simulink model "BBK_client_2006b"  (Simulink 6.5)
settings: Solver=ode3  StartTime=0.0  StopTime=Inf  FixedStep=base_dT  MaxStep=0.01  RelTol=1e-3
values from neighbouring files (symbols this model uses):
  base_dT = Simulink.Parameter    [InternetBBKInit.m]
libraries: simulink x1
settings Model: Creator=akshart  LastModifiedBy=me-dspace
settings DebuggingCC: SignalResolutionControl=UseLocalSettings  FcnCallInpInsideContextMsg=Enable All  StrictBusMsg=ErrorLevel1
settings HardwareCC: TargetHWDeviceType=32-bit Generic
settings CodeAppCC: CustomSymbolStrType=$N$R$M_T
settings GRTTargetCC: ExtModeInterfaceLevel=Level1
settings ConfigurationSet: Description=SimMechanics 2G

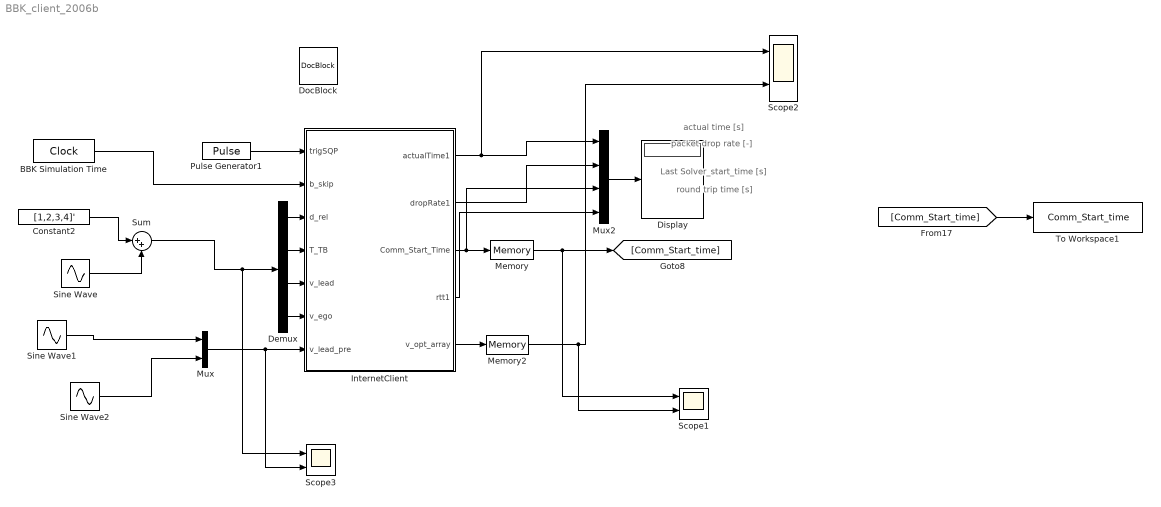
== system BBK_client_2006b ==
  note: actual time [s]
  note: packet drop rate [-]
  note: Last Solver_start_time [s]
  note: round trip time [s]
  BBK Simulation Time : DigitalClock  SampleTime=base_dT
  Constant2 : Constant  Value=[1,2,3,4]'
  Demux : Demux
  Display : Display
  DocBlock : simulink/Model-Wide Utilities/DocBlock  DocumentType=Text
  InternetClient : Subsystem
      mask Type: 20-sim 4.6 S-Function block
      mask Description:
      | This block is generated by the 20-sim Matlab Code Generator.
      | 
      | * look under the mask to get information on the ports
      | * press Help for more detailed information
      | * the parameters of this block are:
      mask Help:
      | This block is generated by the 20-sim Matlab Code Generator<br>
      | The block parameters are:<br><blockquote></blockquote>
      | Generated at:<br>
      | <blockquote><b>date:  </b>June 14, 2017<br>
      | <b>time:  </b>4:16:43 PM<br></blockquote>
      | From the following 20-sim model:<br>
      | <blockquote><b>submodel:  </b>InternetServer<br>
      | <b>model:  </b>export to Simulink - UM<br>
      | <b>file:  </b>C:\Users\Tulga Ersal\Desktop\For Xueru\export to Simulink - UM.emx<br>
      | <b>experiment:  </b>C:\Users\Tulga Ersal\Desktop\For Xueru\export to Simulink - UM.emx<br></blockquote>
      | Using the following 20-sim license:<br>
      | <blockquote><b>user:  </b>The University of Michigan<br>
      | <b>from:  </b>20-sim 4.6 Student License<br>
      | <b>build: </b>4.6.1.6898<br></blockquote>
  Memory : Memory  InheritSampleTime=on  LinearizeAsDelay=on
  Memory2 : Memory  X0=zeros(2,1)  InheritSampleTime=on  LinearizeAsDelay=on
  Mux : Mux  Inputs=2
  Mux2 : Mux
  Pulse Generator1 : DiscretePulseGenerator  PulseType=Time based  Period=1  PulseWidth=20  SampleTime=base_dT
  Scope1 : Scope  NumInputPorts=2
      settings: YMin=-0.25~-0.5  YMax=2.25~4.5
  Scope2 : Scope  NumInputPorts=2
      settings: YMin=-3.575~-5  YMax=32.175~5
  Scope3 : Scope  NumInputPorts=2
      settings: YMin=-1.71028~-1.71028  YMax=15.39249~15.39249  SaveName=ScopeData2
  Sine Wave : Sin  SampleTime=0
  Sine Wave1 : Sin  Amplitude=2  SampleTime=0
  Sine Wave2 : Sin  Amplitude=4  Frequency=2  SampleTime=0
  Sum : Sum  Inputs=|++
  To Workspace1 : ToWorkspace  VariableName=Comm_Start_time  SampleTime=-1  SaveFormat=Structure With Time
  wires:
  Constant2/1 -> Sum/1
  InternetClient/3(Comm_Start_Time) -> Mux2/3, Memory/1
  Memory/1 -> Scope1/1, [Comm_Start_time]
  InternetClient/5(v_opt_array) -> Memory2/1
  Pulse Generator1/1 -> InternetClient/1(trigSQP)
  InternetClient/1(actualTime1) -> Scope2/1, Mux2/1
  InternetClient/2(dropRate1) -> Mux2/2
  InternetClient/4(rtt1) -> Mux2/4
  Mux2/1 -> Display/1
  [Comm_Start_time] -> To Workspace1/1
  Memory2/1 -> Scope1/2, Scope2/2
  BBK Simulation Time/1 -> InternetClient/2(b_skip)
  Mux/1 -> Scope3/2, InternetClient/7(v_lead_pre)
  Sine Wave/1 -> Sum/2
  Demux/1 -> InternetClient/3(d_rel)
  Demux/2 -> InternetClient/4(T_TB)
  Demux/3 -> InternetClient/5(v_lead)
  Demux/4 -> InternetClient/6(v_ego)
  Sum/1 -> Scope3/1, Demux/1
  Sine Wave2/1 -> Mux/2
  Sine Wave1/1 -> Mux/1

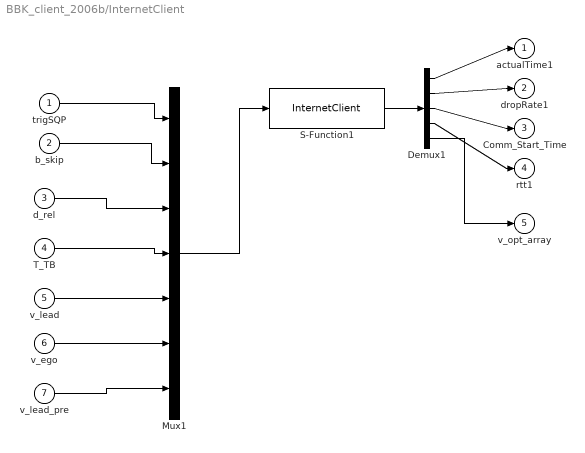
== system BBK_client_2006b/InternetClient ==
  trigSQP : Inport
  b_skip : Inport  Port=2
  d_rel : Inport  Port=3
  T_TB : Inport  Port=4
  v_lead : Inport  Port=5
  v_ego : Inport  Port=6
  v_lead_pre : Inport  Port=7
  Demux1 : Demux  Outputs=[1 1 1 1 2 ]
  Mux1 : Mux  Inputs=[1 1 1 1 1 1 2 ]
  S-Function1 : S-Function  FunctionName=InternetClient  EnableBusSupport=off
  actualTime1 : Outport
  dropRate1 : Outport  Port=2
  Comm_Start_Time : Outport  Port=3
  rtt1 : Outport  Port=4
  v_opt_array : Outport  Port=5
  wires:
  Demux1/1 -> actualTime1/1
  Demux1/2 -> dropRate1/1
  Demux1/3 -> Comm_Start_Time/1
  Demux1/4 -> rtt1/1
  S-Function1/1 -> Demux1/1
  trigSQP/1 -> Mux1/1
  b_skip/1 -> Mux1/2
  Mux1/1 -> S-Function1/1
  T_TB/1 -> Mux1/4
  d_rel/1 -> Mux1/3
  v_lead/1 -> Mux1/5
  v_ego/1 -> Mux1/6
  v_lead_pre/1 -> Mux1/7
  Demux1/5 -> v_opt_array/1
